simulink model "Car13WithRaspPins"  (R2024a)
settings: Solver=FixedStepAuto  StartTime=0.0  StopTime=inf  RelTol=1e-3  EnableMultiTasking=on
model workspace (MAT data in the model file):
  indicator = -1
libraries: raspberrypiBasiclib x9
settings Model: Creator=thipp  LastModifiedBy=thipp
settings SolverCC: PositivePriorityOrder=on
settings OptimizationCC: EnhancedBackFolding=on  PassReuseOutputArgsAs=Individual arguments  ZeroExternalMemoryAtStartup=off  ZeroInternalMemoryAtStartup=off  MaxStackSize=64  OptimizeBlockOrder=speed  DifferentSizesBufferReuse=on  OptimizationCustomize=off  EfficientTunableParamExpr=on
settings DebuggingCC: ParameterTunabilityLossMsg=error
settings HardwareCC: ProdBitPerPointer=32  ProdBitPerSizeT=32  ProdBitPerPtrDiffT=32  ProdLargestAtomicInteger=Long  ProdLargestAtomicFloat=Double  ProdWordSize=32  ProdLongLongMode=on  ProdHWDeviceType=ARM Compatible->ARM Cortex
settings RTWCC: Description=Embedded Coder  SystemTargetFile=ert.tlc  HardwareBoard=Raspberry Pi  TLCOptions="-aInlineSetEventsForThisBaseRateFcn=TLC_FALSE -aSuppressMultiTaskScheduler=TLC_FALSE  -aRateBasedStepFcn=0"  TemplateMakefile=ert_default_tmf  Toolchain=GNU GCC Embedded Linux  BuildConfiguration=Faster Runs
settings CodeAppCC: ForceParamTrailComments=on  IgnoreCustomStorageClasses=off  OperatorAnnotations=on  SimulinkDataObjDesc=on  SFDataObjDesc=on  InsertBlockDesc=on
settings ERTTargetCC: SupportContinuousTime=on  SupportVariableSizeSignals=on  ExtModeTransport=2  ExtModeStaticAlloc=on  ExtModeMexFile=ext_xcp  ExtModeIntrfLevel=Level2 - Open

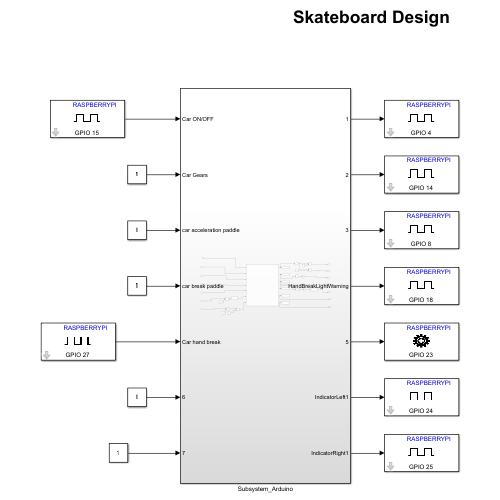
[thumbnail: Simulink's stored preview of the top-level diagram]
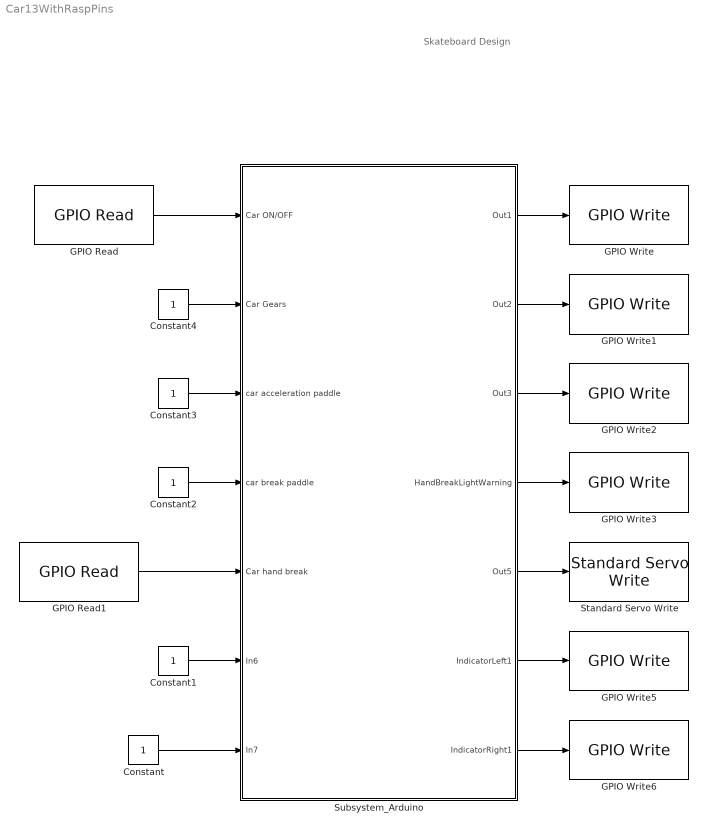
== system Car13WithRaspPins ==
  note: Skateboard Design
  Constant{,1..4} (5 alike) : Constant
  GPIO Read : raspberrypiBasiclib/GPIO Read  board=Model B+  gpio=15  internalResistor=Off  sampleTime=0.1  direction=Input  blockPlatform=Raspberry Pi
  GPIO Read1 : raspberrypiBasiclib/GPIO Read  board=Model B+  gpio=27  internalResistor=Off  sampleTime=0.1  direction=Input  blockPlatform=Raspberry Pi
  GPIO Write : raspberrypiBasiclib/GPIO Write  board=Model B+  gpio=4  direction=Output  blockPlatform=Raspberry Pi
  GPIO Write1 : raspberrypiBasiclib/GPIO Write  board=Model B+  gpio=14  direction=Output  blockPlatform=Raspberry Pi
  GPIO Write2 : raspberrypiBasiclib/GPIO Write  board=Model B+  gpio=8  direction=Output  blockPlatform=Raspberry Pi
  GPIO Write3 : raspberrypiBasiclib/GPIO Write  board=Model B+  gpio=18  direction=Output  blockPlatform=Raspberry Pi
  GPIO Write5 : raspberrypiBasiclib/GPIO Write  board=Model B+  gpio=24  direction=Output  blockPlatform=Raspberry Pi
  GPIO Write6 : raspberrypiBasiclib/GPIO Write  board=Model B+  gpio=25  direction=Output  blockPlatform=Raspberry Pi
  Standard Servo Write : raspberrypiBasiclib/Standard Servo Write  board=Pi 2 Model B  Pin_=23  MinPulseDuration=1000e-6  MaxPulseDuration=2000e-6  blockPlatform=Raspberry Pi
  Subsystem_Arduino : Subsystem
  wires:
  GPIO Read/1 -> Subsystem_Arduino/1(Car ON/OFF)
  Constant4/1 -> Subsystem_Arduino/2(Car Gears)
  Constant3/1 -> Subsystem_Arduino/3(car acceleration paddle)
  Constant2/1 -> Subsystem_Arduino/4(car break paddle)
  GPIO Read1/1 -> Subsystem_Arduino/5("Car hand break ")
  Constant1/1 -> Subsystem_Arduino/6(In6)
  Constant/1 -> Subsystem_Arduino/7(In7)
  Subsystem_Arduino/1(Out1) -> GPIO Write/1
  Subsystem_Arduino/2(Out2) -> GPIO Write1/1
  Subsystem_Arduino/3(Out3) -> GPIO Write2/1
  Subsystem_Arduino/4(HandBreakLightWarning) -> GPIO Write3/1
  Subsystem_Arduino/5(Out5) -> Standard Servo Write/1
  Subsystem_Arduino/6(IndicatorLeft1) -> GPIO Write5/1
  Subsystem_Arduino/7(IndicatorRight1) -> GPIO Write6/1

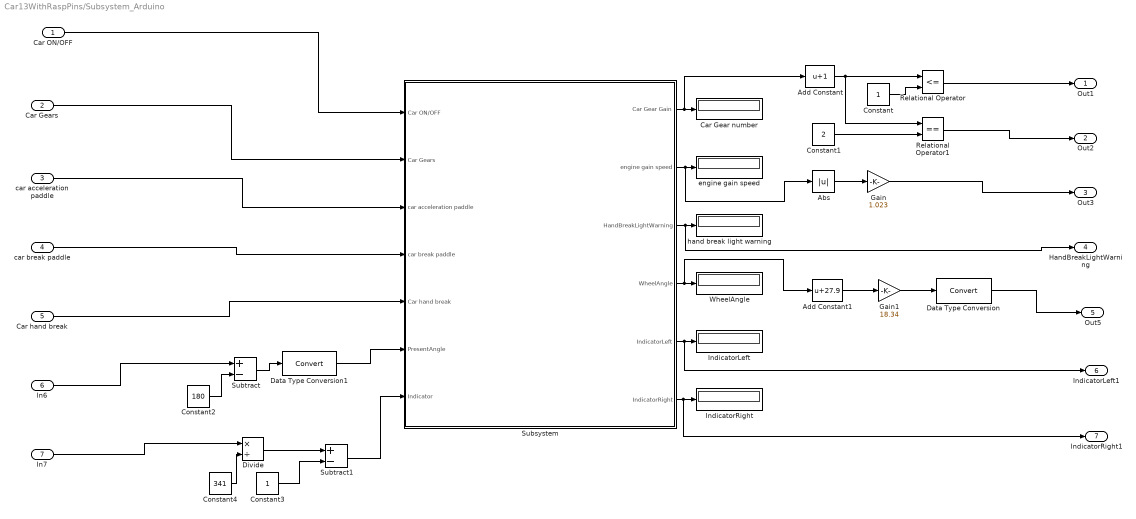
== system Car13WithRaspPins/Subsystem_Arduino ==
  Car ON/OFF : Inport
  Car Gears : Inport  Port=2
  car acceleration paddle : Inport  Port=3
  car break paddle : Inport  Port=4
  "Car hand break " : Inport  Port=5
  In6 : Inport  Port=6
  In7 : Inport  Port=7
  Abs : Abs  SaturateOnIntegerOverflow=off
  Add Constant : Bias  Bias=1  SaturateOnIntegerOverflow=off
  Add Constant1 : Bias  Bias=27.9  SaturateOnIntegerOverflow=off
  Car Gear number : Display
  Constant : Constant
  Constant1 : Constant  Value=2
  Constant2 : Constant  Value=180
  Constant3 : Constant
  Constant4 : Constant  Value=341
  Data Type Conversion : DataTypeConversion  RndMeth=Ceiling  SaturateOnIntegerOverflow=off
  Data Type Conversion1 : DataTypeConversion  SaturateOnIntegerOverflow=off  RndMeth=Floor
  Divide : Product  Inputs=*/
  Gain : Gain  Gain=1.023
  Gain1 : Gain  Gain=18.34
  IndicatorLeft : Display
  IndicatorRight : Display
  Relational Operator : RelationalOperator  Operator=<=  OutDataTypeStr=boolean  RndMeth=Simplest  InputSameDT=off
  Relational Operator1 : RelationalOperator  Operator===  OutDataTypeStr=boolean  RndMeth=Simplest  InputSameDT=off
  Subsystem : Subsystem
  Subtract : Sum  Inputs=+-
  Subtract1 : Sum  Inputs=+-
  WheelAngle : Display
  engine gain speed : Display
  hand break light warning : Display
  Out1 : Outport
  Out2 : Outport  Port=2
  Out3 : Outport  Port=3
  HandBreakLightWarning : Outport  Port=4
  Out5 : Outport  Port=5
  IndicatorLeft1 : Outport  Port=6
  IndicatorRight1 : Outport  Port=7
  wires:
  Divide/1 -> Subtract1/1
  Subsystem/3(HandBreakLightWarning) -> HandBreakLightWarning/1, hand break light warning/1
  Car ON/OFF/1 -> Subsystem/1(Car ON/OFF)
  Subsystem/4(WheelAngle) -> Add Constant1/1, WheelAngle/1
  Subsystem/2(engine gain speed) -> Abs/1, engine gain speed/1
  Subsystem/1(Car Gear Gain) -> Add Constant/1, Car Gear number/1
  Constant4/1 -> Divide/2
  Subsystem/6(IndicatorRight) -> IndicatorRight1/1, IndicatorRight/1
  Subsystem/5(IndicatorLeft) -> IndicatorLeft1/1, IndicatorLeft/1
  Car Gears/1 -> Subsystem/2(Car Gears)
  Subtract/1 -> Data Type Conversion1/1
  Subtract1/1 -> Subsystem/7(Indicator)
  Add Constant1/1 -> Gain1/1
  Relational Operator1/1 -> Out2/1
  Constant3/1 -> Subtract1/2
  In7/1 -> Divide/1
  Gain/1 -> Out3/1
  Add Constant/1 -> Relational Operator1/1, Relational Operator/1
  Constant/1 -> Relational Operator/2
  Constant1/1 -> Relational Operator1/2
  In6/1 -> Subtract/1
  car break paddle/1 -> Subsystem/4(car break paddle)
  Gain1/1 -> Data Type Conversion/1
  Abs/1 -> Gain/1
  Relational Operator/1 -> Out1/1
  Data Type Conversion1/1 -> Subsystem/6(PresentAngle)
  car acceleration paddle/1 -> Subsystem/3(car acceleration paddle)
  Constant2/1 -> Subtract/2
  "Car hand break "/1 -> Subsystem/5("Car hand break ")
  Data Type Conversion/1 -> Out5/1

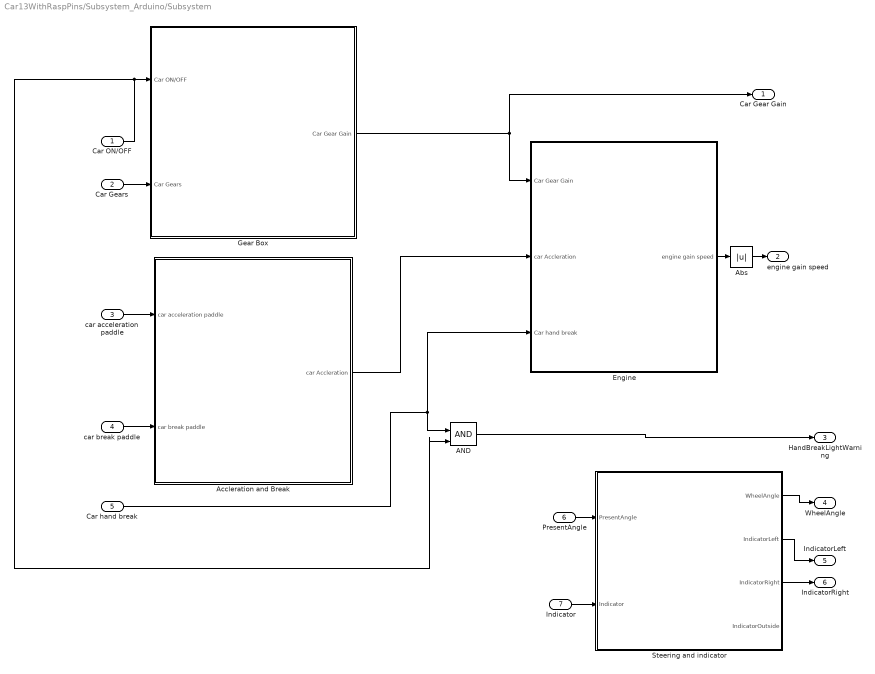
== system Car13WithRaspPins/Subsystem_Arduino/Subsystem ==
  Car ON/OFF : Inport
  Car Gears : Inport  Port=2
  car acceleration paddle : Inport  Port=3
  car break paddle : Inport  Port=4
  "Car hand break " : Inport  Port=5
  PresentAngle : Inport  Port=6
  Indicator : Inport  Port=7
  AND : Logic  IconShape=distinctive  AllPortsSameDT=off  OutDataTypeStr=boolean
  Abs : Abs  SaturateOnIntegerOverflow=off
  Accleration and Break : Subsystem
  Engine : Subsystem
  Gear Box : Subsystem
  "Steering and indicator " : Subsystem
  Car Gear Gain : Outport
  engine gain speed : Outport  Port=2
  HandBreakLightWarning : Outport  Port=3
  WheelAngle : Outport  Port=4
  IndicatorLeft : Outport  Port=5
  IndicatorRight : Outport  Port=6
  wires:
  Gear Box/1(Car Gear Gain) -> Engine/1(Car Gear Gain), Car Gear Gain/1
  Car ON/OFF/1 -> Gear Box/1(Car ON/OFF), AND/2
  Accleration and Break/1(car Accleration) -> Engine/2(car Accleration)
  "Steering and indicator "/3(IndicatorRight) -> IndicatorRight/1
  "Steering and indicator "/2(IndicatorLeft) -> IndicatorLeft/1
  car acceleration paddle/1 -> Accleration and Break/1(car acceleration paddle)
  Indicator/1 -> "Steering and indicator "/2(Indicator)
  "Car hand break "/1 -> Engine/3("Car hand break "), AND/1
  Engine/1(engine gain speed) -> Abs/1
  car break paddle/1 -> Accleration and Break/2(car break paddle)
  Car Gears/1 -> Gear Box/2(Car Gears)
  Abs/1 -> engine gain speed/1
  "Steering and indicator "/1(WheelAngle) -> WheelAngle/1
  AND/1 -> HandBreakLightWarning/1
  PresentAngle/1 -> "Steering and indicator "/1(PresentAngle)

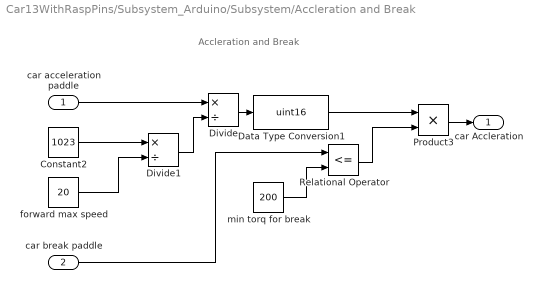
== system Car13WithRaspPins/Subsystem_Arduino/Subsystem/Accleration and Break ==
  note: Accleration and Break
  car acceleration paddle : Inport
  car break paddle : Inport  Port=2
  Constant2 : Constant  Value=1023
  Data Type Conversion1 : DataTypeConversion  OutDataTypeStr=uint16  SaturateOnIntegerOverflow=off  RndMeth=Floor
  Divide : Product  Inputs=*/  RndMeth=Zero  SaturateOnIntegerOverflow=on
  Divide1 : Product  Inputs=*/  RndMeth=Zero  SaturateOnIntegerOverflow=on
  Product3 : Product
  Relational Operator : RelationalOperator  Operator=<=  OutDataTypeStr=boolean  RndMeth=Simplest  InputSameDT=off
  forward max speed : Constant  Value=20
  min torq for break : Constant  Value=200
  car Accleration : Outport
  wires:
  min torq for break/1 -> Relational Operator/2
  Divide/1 -> Data Type Conversion1/1
  forward max speed/1 -> Divide1/2
  car break paddle/1 -> Relational Operator/1
  Data Type Conversion1/1 -> Product3/1
  Constant2/1 -> Divide1/1
  Divide1/1 -> Divide/2
  Relational Operator/1 -> Product3/2
  car acceleration paddle/1 -> Divide/1
  Product3/1 -> car Accleration/1

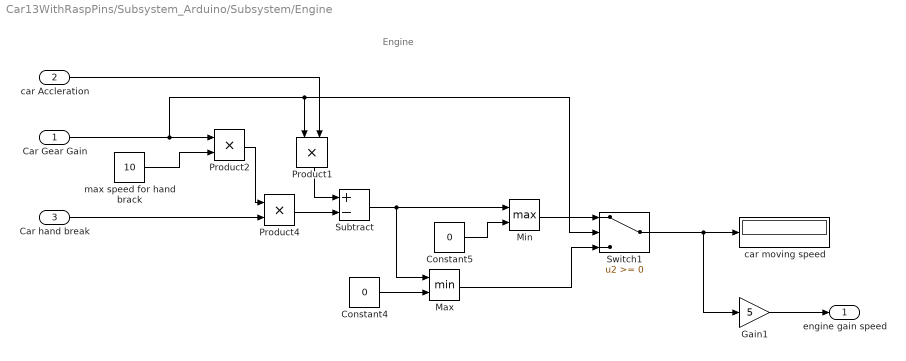
== system Car13WithRaspPins/Subsystem_Arduino/Subsystem/Engine ==
  note: Engine
  Car Gear Gain : Inport
  car Accleration : Inport  Port=2
  "Car hand break " : Inport  Port=3
  Constant4 : Constant  Value=0
  Constant5 : Constant  Value=0
  Gain1 : Gain  Gain=5
  Max : MinMax  Inputs=2
  Min : MinMax  Function=max  Inputs=2
  Product1 : Product
  Product2 : Product
  Product4 : Product
  Subtract : Sum  Inputs=+-
  Switch1 : Switch  SaturateOnIntegerOverflow=off  InputSameDT=off
  car moving speed : Display
  max speed for hand brack : Constant  Value=10
  engine gain speed : Outport
  wires:
  Subtract/1 -> Min/1, Max/1
  Switch1/1 -> Gain1/1, car moving speed/1
  Product2/1 -> Product4/1
  Product1/1 -> Subtract/1
  Product4/1 -> Subtract/2
  Constant5/1 -> Min/2
  max speed for hand brack/1 -> Product2/2
  Car Gear Gain/1 -> Product1/1, Switch1/2, Product2/1
  Max/1 -> Switch1/3
  Min/1 -> Switch1/1
  Constant4/1 -> Max/2
  car Accleration/1 -> Product1/2
  "Car hand break "/1 -> Product4/2
  Gain1/1 -> engine gain speed/1

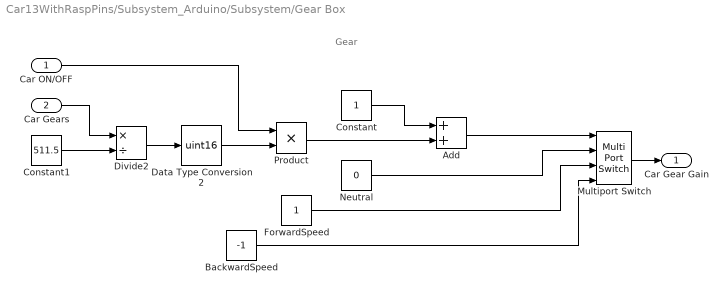
== system Car13WithRaspPins/Subsystem_Arduino/Subsystem/Gear Box ==
  note: Gear
  Car ON/OFF : Inport
  Car Gears : Inport  Port=2
  Add : Sum
  BackwardSpeed : Constant  Value=-1
  Constant : Constant
  Constant1 : Constant  Value=511.5
  Data Type Conversion2 : DataTypeConversion  OutDataTypeStr=uint16  RndMeth=Nearest  SaturateOnIntegerOverflow=off
  Divide2 : Product  Inputs=*/  RndMeth=Zero  SaturateOnIntegerOverflow=on
  ForwardSpeed : Constant
  Multiport Switch : MultiPortSwitch  SaturateOnIntegerOverflow=off  InputSameDT=off
  Neutral : Constant  Value=0
  Product : Product
  Car Gear Gain : Outport
  wires:
  Add/1 -> Multiport Switch/1
  Neutral/1 -> Multiport Switch/2
  Constant1/1 -> Divide2/2
  Product/1 -> Add/2
  BackwardSpeed/1 -> Multiport Switch/4
  Data Type Conversion2/1 -> Product/2
  ForwardSpeed/1 -> Multiport Switch/3
  Divide2/1 -> Data Type Conversion2/1
  Constant/1 -> Add/1
  Car Gears/1 -> Divide2/1
  Multiport Switch/1 -> Car Gear Gain/1
  Car ON/OFF/1 -> Product/1

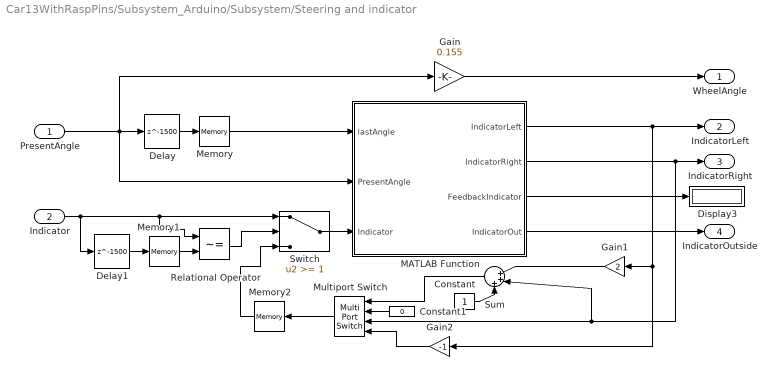
== system Car13WithRaspPins/Subsystem_Arduino/Subsystem/Steering and indicator  ==
  PresentAngle : Inport
  Indicator : Inport  Port=2
  Constant : Constant
  Constant1 : Constant  Value=0
  Delay : Delay  DelayLength=1500
  Delay1 : Delay  DelayLength=1500
  Display3 : Display
  Gain : Gain  Gain=0.155
  Gain1 : Gain  Gain=2
  Gain2 : Gain  Gain=-1
  MATLAB Function : MATLAB Function  TreatAsAtomicUnit=on
  Memory : Memory
  Memory1 : Memory
  Memory2 : Memory
  Multiport Switch : MultiPortSwitch  SaturateOnIntegerOverflow=off  InputSameDT=off
  Relational Operator : RelationalOperator  Operator=~=  OutDataTypeStr=boolean  RndMeth=Simplest  InputSameDT=off
  Sum : Sum  Inputs=|+++
  Switch : Switch  Threshold=1  SaturateOnIntegerOverflow=off  InputSameDT=off
  WheelAngle : Outport
  IndicatorLeft : Outport  Port=2
  IndicatorRight : Outport  Port=3
  IndicatorOutside : Outport  Port=4
  wires:
  PresentAngle/1 -> MATLAB Function/2(PresentAngle), Gain/1, Delay/1
  MATLAB Function/1(IndicatorLeft) -> Gain2/1, Gain1/1, IndicatorLeft/1
  Gain/1 -> WheelAngle/1
  MATLAB Function/3(FeedbackIndicator) -> Display3/1
  Memory/1 -> MATLAB Function/1(lastAngle)
  Delay/1 -> Memory/1
  MATLAB Function/4(IndicatorOut) -> IndicatorOutside/1
  Indicator/1 -> Delay1/1, Relational Operator/1, Switch/1
  Relational Operator/1 -> Switch/2
  Switch/1 -> MATLAB Function/3(Indicator)
  Memory1/1 -> Relational Operator/2
  Delay1/1 -> Memory1/1
  Memory2/1 -> Switch/3
  Sum/1 -> Multiport Switch/1
  Constant/1 -> Sum/3
  Constant1/1 -> Multiport Switch/2
  MATLAB Function/2(IndicatorRight) -> Sum/2, Multiport Switch/3, IndicatorRight/1
  Gain1/1 -> Sum/1
  Gain2/1 -> Multiport Switch/4
  Multiport Switch/1 -> Memory2/1

== matlab function Car13WithRaspPins/Subsystem_Arduino/Subsystem/Steering and indicator /MATLAB Function ==
  data: IndicatorLeft output; IndicatorRight output; FeedbackIndicator output; IndicatorOut output; lastAngle input; PresentAngle input; Indicator input
function [IndicatorLeft, IndicatorRight,FeedbackIndicator,IndicatorOut] = fcn(lastAngle, PresentAngle, Indicator)
    % Determine the turning direction
    turning = 0;
    if PresentAngle> lastAngle 
        turning = 1; % Turning right
    elseif PresentAngle< lastAngle 
        turning = -1; % Turning left
    end
    
    % Update the indicator position based on the turning direction
    IndicatorPosition = Indicator;
    if Indicator == 1 && turning == -1
        IndicatorPosition = 0; % Cancel right indicator when turning left
    elseif Indicator == -1 && turning == 1
        IndicatorPosition = 0; % Cancel left indicator when turning right
    end
    
    % Determine the state of left and right indicators
    LI = 0;
    RI = 0;
    FB = 0;
    if IndicatorPosition == -1
        LI = 1; % Left indicator is on
        FB=-1;
    end
    if IndicatorPosition == 1
        RI = 1; % Right indicator is on
        FB=1;
    end
    
    % Assign outputs
    IndicatorOut = IndicatorPosition;
    IndicatorLeft = LI;
    IndicatorRight = RI;
    FeedbackIndicator = FB;
end
